simulink model "Current_Macchina3DOF"  (R2023a)
settings: Solver=VariableStepAuto  StartTime=0.0  StopTime=100  RelTol=1e-3
model workspace (MAT data in the model file):
  EngPwr = 352122.842504
  EngWc = 4.047
  Tdiff = 849
  Tlim = 1000
  VEH.Mass = 1181
  VEH.StaticNormalFrontLoad.FR = 264.666666667
  VEH.StaticNormalFrontLoad.FL = 264.666666667
  VEH.StaticNormalRearLoad.RR = 322
  VEH.StaticNormalRearLoad.RL = 322
  VEH.WheelBase = 3.075
  VEH.FrontAxlePositionfromCG = 1.515
  VEH.RearAxlePositionfromCG = 1.504
  VEH.HeightCG = 0.134
  VEH.FrontalArea = 2.11
  VEH.DragCoefficient = 0.33
  VEH.NumberOfWheelsPerAxle = 2
  VEH.Thread.FR = 1.705
  VEH.Thread.RR = 1.705
  VEH.PitchMomentInertia = 1922.66666667
  VEH.RollMomentInertia = 432.333333333
  VEH.YawMomentInertia = 2066
  VEH.SteeringRatio = 18
  VEH.TrackWidth = 1.922
  VEH.SprungMass = 1096.72266667
  VEH.InitialLongPosition = 0
  VEH.InitialLatPosition = 3.125
  VEH.InitialVertPosition = 0.0111
  VEH.InitialRollAngle = 0
  VEH.InitialPitchAngle = -0.000732
  VEH.InitialYawAngle = 0
  VEH.InitialLongVel = 0
  VEH.InitialLatVel = 0
  VEH.InitialVertVel = 0
  VEH.InitialRollRate = 0
  VEH.InitialPitchRate = 0
  VEH.InitialYawRate = 0
libraries: vehdynlibtirecommon x4, sim3dphyssensorlib x4, autolibutils x3, visionsinks x3, sim3dcameralib x2, sharedtransform x2, vehdynlibsteering x2, vehdynlibtire x1, sim3dlib x1, vdynlib x1, autolibshared x1
settings Model: Creator=gabri  LastModifiedBy=Luzi

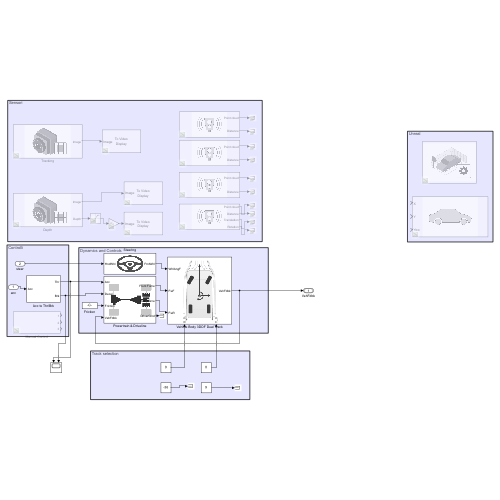
[thumbnail: Simulink's stored preview of the top-level diagram]
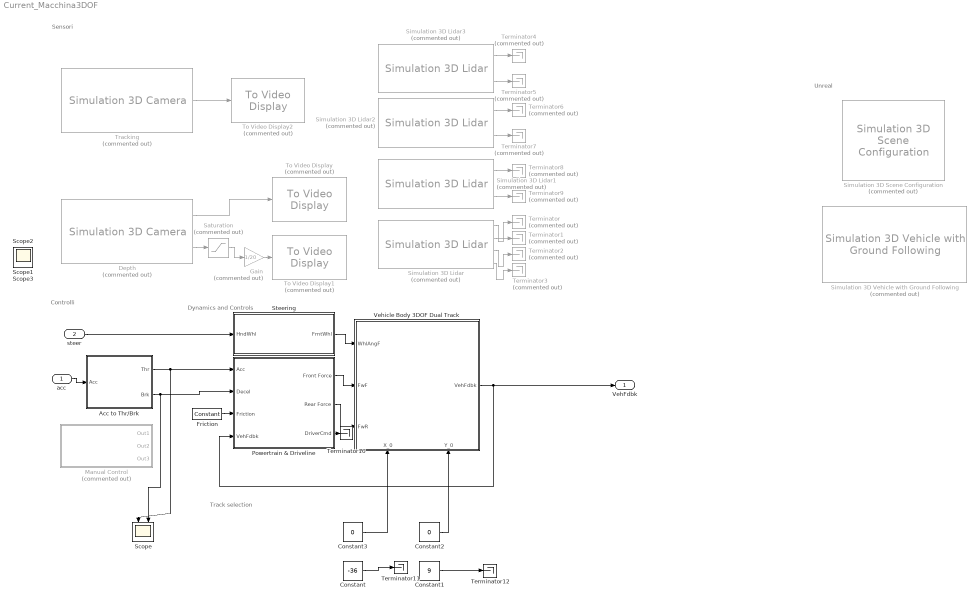
== system Current_Macchina3DOF ==
  note: Track selection
  note: Controlli
  note: Sensori
  note: Unreal
  note: Dynamics and Controls
  acc : Inport  LockScale=on
  steer : Inport  Port=2
  Acc to Thr/Brk : Subsystem
  Constant : Constant  Value=-36
  Constant1 : Constant  Value=9
  Constant2 : Constant  Value=0
  Constant3 : Constant  Value=0
  Depth : sim3dcameralib/Simulation 3D Camera  Priority=1  Commented=on  sensorTag=Sim3dSensor1  sensorId=1  sensorName=Sim3dSensor1  vehTagList={'Scene Origin';'SimulinkVehicle1'}  vehTag=SimulinkVehicle1  mountLoc=Origin  offsetFlag=on  tmountOffset=[-0.236, -0.01, 1.265]  extTmount=off  rmountOffset=[0, 0, 0]  extRmount=off  FocalLength=[643, 643]  OpticalCenter=[640, 360]  ImageSize=[720, 1280]  RadialDistortion=[0, 0]  TangentialDistortion=[0, 0]  SensorSkew=0  DepthOutportEnabled=on  SemanticOutportEnabled=off  TransformOutportEnabled=off  SampleTime=-1  mountPoint=[-0.236 0.01 1.265]  mountOrientation=[0 0 0]  aMode=3  ID=1
      settings: LibrarySourceBlock=drivingsim3d/Simulation 3D Camera
  Friction : vehdynlibtirecommon/Constant  const=0.8  numWheels=4
  Gain : Gain  Commented=on  Gain=1/20
  Manual Control : Subsystem  Commented=on
  Powertrain & Driveline : Subsystem
      mask Display: image('vdbslibpt.png');
  Saturation : Saturate  Commented=on  UpperLimit=20  LowerLimit=0
  Scope : Scope  NumInputPorts=2
  Simulation 3D Lidar : sim3dphyssensorlib/Simulation 3D Lidar  Priority=1  Commented=on  sensorTag=Sim3dSensor3  sensorId=3  sensorName=Sim3dSensor3  vehTagList={'Scene Origin';'SimulinkVehicle1'}  vehTag=SimulinkVehicle1  mountLoc=Origin  offsetFlag=on  tmountOffset=[1.52, -0.348, 0.12]  rmountOffset=[0, 0, 0]  DetectionRange=12  RangeResolution=0.01  VerticalFOV=2  VerticalResolution=2  HorizontalFOV=2  HorizontalResolution=0.54  DistanceOutportEnabled=on  ReflectivityOutportEnabled=off  SemanticOutportEnabled=off  TransformOutportEnabled=on  SampleTime=-1  mountPoint=[1.52 0.348 0.12]  mountOrientation=[0 0 0]  aMode=3  ID=3
      settings: LibrarySourceBlock=drivingsim3d/Simulation 3D Lidar
  Simulation 3D Lidar1 : sim3dphyssensorlib/Simulation 3D Lidar  Priority=1  Commented=on  sensorTag=Sim3dSensor4  sensorId=4  sensorName=Sim3dSensor4  vehTagList={'Scene Origin';'SimulinkVehicle1'}  vehTag=SimulinkVehicle1  mountLoc=Origin  offsetFlag=on  tmountOffset=[1.515, -0.393, 0.12]  rmountOffset=[0, 0, -22]  DetectionRange=12  RangeResolution=0.01  VerticalFOV=2  VerticalResolution=2  HorizontalFOV=2  HorizontalResolution=0.54  DistanceOutportEnabled=on  ReflectivityOutportEnabled=off  SemanticOutportEnabled=off  TransformOutportEnabled=off  SampleTime=-1  mountPoint=[1.515 0.393 0.12]  mountOrientation=[0 0 22]  aMode=3  ID=4
      settings: LibrarySourceBlock=drivingsim3d/Simulation 3D Lidar
  Simulation 3D Lidar2 : sim3dphyssensorlib/Simulation 3D Lidar  Priority=1  Commented=on  sensorTag=Sim3dSensor5  sensorId=5  sensorName=Sim3dSensor5  vehTagList={'Scene Origin';'SimulinkVehicle1'}  vehTag=SimulinkVehicle1  mountLoc=Origin  offsetFlag=on  tmountOffset=[1.52, 0.348, 0.12]  rmountOffset=[0, 0, 0]  DetectionRange=12  RangeResolution=0.01  VerticalFOV=2  VerticalResolution=2  HorizontalFOV=2  HorizontalResolution=0.54  DistanceOutportEnabled=on  ReflectivityOutportEnabled=off  SemanticOutportEnabled=off  TransformOutportEnabled=off  SampleTime=-1  mountPoint=[1.52 -0.348 0.12]  mountOrientation=[0 0 0]  aMode=3  ID=5
      settings: LibrarySourceBlock=drivingsim3d/Simulation 3D Lidar
  Simulation 3D Lidar3 : sim3dphyssensorlib/Simulation 3D Lidar  Priority=1  Commented=on  sensorTag=Sim3dSensor6  sensorId=6  sensorName=Sim3dSensor6  vehTagList={'Scene Origin';'SimulinkVehicle1'}  vehTag=SimulinkVehicle1  mountLoc=Origin  offsetFlag=on  tmountOffset=[1.515, 0.393, 0.12]  rmountOffset=[0, 0, 22]  DetectionRange=12  RangeResolution=0.01  VerticalFOV=2  VerticalResolution=2  HorizontalFOV=2  HorizontalResolution=0.54  DistanceOutportEnabled=on  ReflectivityOutportEnabled=off  SemanticOutportEnabled=off  TransformOutportEnabled=off  SampleTime=-1  mountPoint=[1.515 -0.393 0.12]  mountOrientation=[0 0 -22]  aMode=3  ID=6
      settings: LibrarySourceBlock=drivingsim3d/Simulation 3D Lidar
  Simulation 3D Scene Configuration : sim3dlib/Simulation 3D Scene Configuration  Priority=0  Commented=on  ProjectFormat=Unreal Editor  SceneDesc=Straight road  ProjectName=D:\MATLAB\toolbox\shared\sim3d_projects\automotive_project\UE4\WindowsNoEditor\VehicleSimulation.exe  ScenePath=/Game/Maps/HwStrght  UEProjPath=C:\Users\gabriele\Documents\Unreal Projects\4_27\FSAE\RT3D\RT3D.uproject  EnableOpenDRIVE=off  vehTagList={'Scene Origin';'SimulinkVehicle1'}  vehTag=SimulinkVehicle1  OpVisEn=off  Ts=.01  EnableWindow=on  EnableRemoteAccess=off  EnableWeather=off  SunAltitude=40.0  SunAzimuth=90  clouds=10  wind=1  fog=0  rain=0  EnableGeospatial=off  OriginHeight=200  OriginLatitude=40.744652  OriginLongitude=-73.988864  MapStyle=Aerial  AdditionalAssetIDs=[]  UseAdvancedSunSky=off  SolarTime=11  TimeZone=-5  Day=21  Month=9  Year=2022  UseDaylightSavingTime=on  DSTStartDay=10  DSTStartMonth=3  DSTEndDay=3  DSTEndMonth=11  DSTSwitchHour=2  sensorTag=MainCamera1  sensorId=1  sensorName=MainCamera1  mountLoc=Origin  offsetFlag=off  tmountOffset=[0, 0, 0]  rmountOffset=[0, 0, 0]  HorizontalResolution=1280  VerticalResolution=720  HorizontalFOV=60  mountPoint=[0 0 0]  mountOrientation=[0 0 0]  aMode=2  ID=1  GeoTrigger=Inactive
      settings: LibrarySourceBlock=vdynlib/Vehicle Scenarios/Sim3D/Sim3D Core/Simulation 3D Scene Configuration
  Simulation 3D Vehicle with Ground Following : vdynlib/Vehicle Scenarios/Sim3D/Sim3D Vehicle/Components/Simulation 3D Vehicle with Ground Following  Priority=-1  Commented=on  PassVehMesh=Custom  MeshPath=/Game/Car1/FC_Model.FC_Model  TrackWidth=1.4  WheelBase=3  WheelRadius=0.35  VehColor=Red  InitialPos=[0, 0, 0]  InitialRot=[0, 0, 0]  ActorName=SimulinkVehicle1  VehLightsControl=off  HeadlightColor=[ 1, 1, 1 ]  HighBeamIntensity=100000  LowBeamIntensity=60000  HighBeamConeAngle=1.22  LowBeamConeAngle=1.22  LeftHeadlightOrientation=[ 0, 0 ]  RightHeadlightOrientation=[ 0, 0 ]  BrakelightIntensity=200  ReverselightIntensity=500  SignallightIntensity=500  SignallightPeriod=1  SignalPulseWidth=50  SampleTime=-1  ActorType=SimulinkVehicle  ID=1  aMode=2  ActorTag=SimulinkVehicle1  CoordinateScheme=SAE
  Steering : Subsystem
      mask Display: image('vdbslibsteer.png');
  Terminator{,1..9} (10 alike) : Terminator  Commented=on
  Terminator10 : Terminator
  Terminator11 : Terminator
  Terminator12 : Terminator
  To Video Display : visionsinks/To Video Display  Commented=on  windowSizeMode=Normal  openAtMdlStart=on  fullScreen=off  videoWindowX=536805376  videoWindowY=536805376  saveWindowSize=off  videoWindowWidth=2147483647  videoWindowHeight=2147483647  inputColorFormat=RGB  inputType=Obsolete  imagePorts=One multidimensional signal  OutputDevice=On-screen video monitor  dataOrg=Column-major  isWindowOpen=off
  To Video Display1 : visionsinks/To Video Display  Commented=on  windowSizeMode=Normal  openAtMdlStart=on  fullScreen=off  videoWindowX=536805376  videoWindowY=536805376  saveWindowSize=off  videoWindowWidth=2147483647  videoWindowHeight=2147483647  inputColorFormat=RGB  inputType=Obsolete  imagePorts=One multidimensional signal  OutputDevice=On-screen video monitor  dataOrg=Column-major  isWindowOpen=off
  To Video Display2 : visionsinks/To Video Display  Commented=on  windowSizeMode=Normal  openAtMdlStart=on  fullScreen=off  videoWindowX=536805376  videoWindowY=536805376  saveWindowSize=off  videoWindowWidth=2147483647  videoWindowHeight=2147483647  inputColorFormat=RGB  inputType=Obsolete  imagePorts=One multidimensional signal  OutputDevice=On-screen video monitor  dataOrg=Column-major  isWindowOpen=off
  Tracking : sim3dcameralib/Simulation 3D Camera  Priority=1  Commented=on  sensorTag=Sim3dSensor2  sensorId=2  sensorName=Sim3dSensor2  vehTagList={'Scene Origin';'SimulinkVehicle1'}  vehTag=SimulinkVehicle1  mountLoc=Origin  offsetFlag=on  tmountOffset=[0.855, 0, 0.655]  extTmount=off  rmountOffset=[0, 0, 0]  extRmount=off  FocalLength=[643, 643]  OpticalCenter=[640, 360]  ImageSize=[720, 1280]  RadialDistortion=[0, 0]  TangentialDistortion=[0, 0]  SensorSkew=0  DepthOutportEnabled=off  SemanticOutportEnabled=off  TransformOutportEnabled=off  SampleTime=-1  mountPoint=[0.855 0 0.655]  mountOrientation=[0 0 0]  aMode=3  ID=2
      settings: LibrarySourceBlock=drivingsim3d/Simulation 3D Camera
  Vehicle Body 3DOF Dual Track : Subsystem
      settings: PortSchema="{\"entries\":[{\"content\":{\"sides\":[{\"content\":{\"connectorIds\":[\"In1\",\"In2\",\"In3\"]},\"type\":\"ConnectorPlacement.EquallySpacedRectSide\",\"uuid\":\"4036215f-6a7b-43f4-bf3a-9e74b907d558\"},{\"content\":{\"connectorIds\":[\"Out1\"],\"side\":\"RIGHT\"},\"type\":\"ConnectorPlacement.EquallySpacedRectSide\",\"uuid\":\"eff6a8c4-1212-4912-9320-06419e317e63\"},{\"content\":{\"side\":\"TOP\"},\"type\":\"ConnectorPlacement.EquallySpacedRectSide\",\"uuid\":\"7c86d461-eb08-4ad0-9f05-3e331398aa8b\"},{\"content\":{\"connectorIds\":[\"In4\",\"In5\"],\"side\":\"BOTTOM\"},\"type\":\"ConnectorPlacement.EquallySpacedRectSide\",\"uuid\":\"b22d0b58-a589-4aa7-a626-c5ccf618b747\"}]},\"type\":\"ConnectorPlacement.EquallySpacedConnector\",\"uuid\":\"19937682-2ace-470e-aa72-0faa8a79652b\"}],\"packageUris\":[\"http://schema.mathworks.com/mf0/Connector/R2020b\"],\"version\":\"1.0\"}"
      mask Display: image('3dofdtrack.png');
  VehFdbk : Outport  OutDataTypeStr=Bus: VehFdbk
  Scope1 : Scope
  Scope2 : Scope
  Scope3 : Scope
  wires:
  Powertrain & Driveline/2(Rear Force) -> Vehicle Body 3DOF Dual Track/3(FwR)
  Steering/1(FrntWhl) -> Vehicle Body 3DOF Dual Track/1(WhlAngF)
  Powertrain & Driveline/1(Front Force) -> Vehicle Body 3DOF Dual Track/2(FwF)
  Friction/1 -> Powertrain & Driveline/3(Friction)
  Depth/2 -> Saturation/1
  Depth/1 -> To Video Display/1
  Saturation/1 -> Gain/1
  Gain/1 -> To Video Display1/1
  Simulation 3D Lidar/1 -> Terminator/1
  Simulation 3D Lidar/2 -> Terminator1/1
  Constant/1 -> Terminator11/1
  Constant1/1 -> Terminator12/1
  Simulation 3D Lidar/3 -> Terminator2/1
  Simulation 3D Lidar/4 -> Terminator3/1
  Constant2/1 -> Vehicle Body 3DOF Dual Track/5(Y_0)
  Tracking/1 -> To Video Display2/1
  Simulation 3D Lidar3/1 -> Terminator4/1
  Simulation 3D Lidar3/2 -> Terminator5/1
  Simulation 3D Lidar2/1 -> Terminator6/1
  Simulation 3D Lidar2/2 -> Terminator7/1
  Simulation 3D Lidar1/1 -> Terminator8/1
  Simulation 3D Lidar1/2 -> Terminator9/1
  Constant3/1 -> Vehicle Body 3DOF Dual Track/4(X_0)
  Vehicle Body 3DOF Dual Track/1(VehFdbk) -> Powertrain & Driveline/4(VehFdbk), VehFdbk/1
  Powertrain & Driveline/3(DriverCmd) -> Terminator10/1
  acc/1 -> Acc to Thr/Brk/1(Acc)
  Acc to Thr/Brk/1(Thr) -> Scope/1, Powertrain & Driveline/1(Acc)
  Acc to Thr/Brk/2(Brk) -> Powertrain & Driveline/2(Decel), Scope/2
  steer/1 -> Steering/1(HndWhl)

== system Current_Macchina3DOF/Acc to Thr//Brk ==
  Acc : Inport
  Switch1 : Switch  Criteria=u2 > Threshold  SaturateOnIntegerOverflow=off  InputSameDT=off
  Switch2 : Switch  Criteria=u2 > Threshold  SaturateOnIntegerOverflow=off  InputSameDT=off
  Unary Minus : UnaryMinus
  Zero : Constant  Value=0  OutDataTypeStr=Inherit: Inherit via back propagation
  Zero1 : Constant  Value=0  OutDataTypeStr=Inherit: Inherit via back propagation
  Thr : Outport
  Brk : Outport  Port=2
  wires:
  Acc/1 -> Switch1/1, Switch1/2, Unary Minus/1, Switch2/2
  Zero1/1 -> Switch1/3
  Switch1/1 -> Thr/1
  Zero/1 -> Switch2/1
  Unary Minus/1 -> Switch2/3
  Switch2/1 -> Brk/1

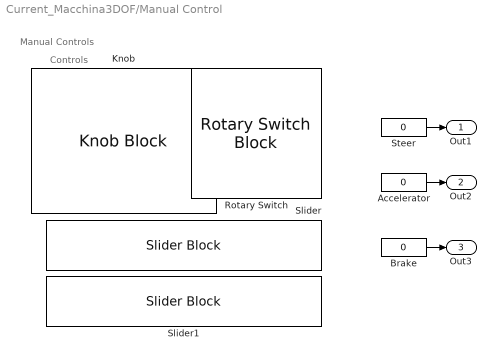
== system Current_Macchina3DOF/Manual Control ==
  note: Manual Controls
  note: Controls
  Accelerator : Constant  Value=0  SampleTime=-1
  Brake : Constant  Value=0  SampleTime=-1
  Knob : KnobBlock  LabelPosition=Bottom  ScaleMin=-90  ScaleMax=90  TickInterval=30
  Rotary Switch : RotarySwitchBlock  LabelPosition=Bottom
      settings: Values={{'R', 'N', 'D'}, [-1 0 1]}
  Slider : SliderBlock  LabelPosition=Bottom  ScaleMax=1  TickInterval=.2
  Slider1 : SliderBlock  LabelPosition=Bottom  ScaleMax=1  TickInterval=.2
  Steer : Constant  Value=0  SampleTime=-1
  Out1 : Outport
  Out2 : Outport  Port=2
  Out3 : Outport  Port=3
  wires:
  Steer/1 -> Out1/1
  Brake/1 -> Out3/1
  Accelerator/1 -> Out2/1

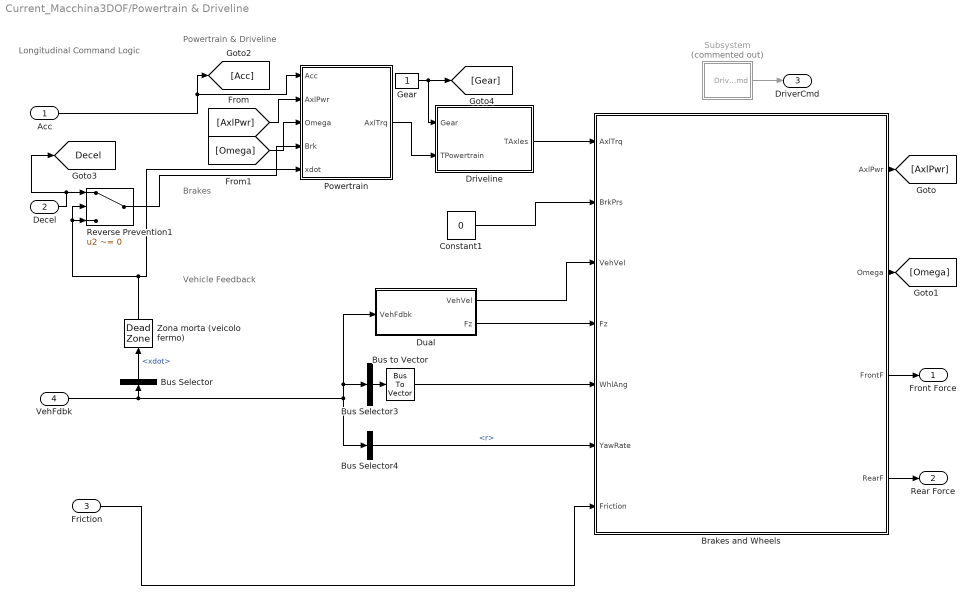
== system Current_Macchina3DOF/Powertrain & Driveline ==
  note: Longitudinal Command Logic
  note: Brakes
  note: Powertrain & Driveline
  note: Vehicle Feedback
  Acc : Inport
  Decel : Inport  Port=2
  Friction : Inport  Port=3
  VehFdbk : Inport  Port=4
  Brakes and Wheels : Subsystem  TreatAsAtomicUnit=on
      mask Display: image('vdbslibwhls.png');
  Bus Selector : BusSelector  OutputSignals=BdyFrm.Cg.Vel.xdot
  Bus Selector3 : BusSelector  OutputSignals=BdyFrm.FrntAxl.Steer.WhlAngFL,BdyFrm.FrntAxl.Steer.WhlAngFR,BdyFrm.RearAxl.Steer.WhlAngRL,BdyFrm.RearAxl.Steer.WhlAngRR  OutputAsBus=on
  Bus Selector4 : BusSelector  OutputSignals=BdyFrm.Cg.AngVel.r
  Bus to Vector : BusToVector
  Constant1 : Constant  Value=0
  Driveline : Subsystem  Variant=on  VariantControlMode=label  VariantControl=Variant1  LabelModeActiveChoice=0
  Dual : Subsystem  VariantControl=1
  Gear : Constant
  Powertrain : Subsystem
  Reverse Prevention1 : Switch  Criteria=u2 ~= 0  SaturateOnIntegerOverflow=off  InputSameDT=off
  Subsystem : Subsystem  Commented=on
  Zona morta (veicolo fermo) : DeadZone  LowerValue=-0.3  UpperValue=0.0002
  Front Force : Outport  VectorParamsAs1DForOutWhenUnconnected=off
  Rear Force : Outport  Port=2  VectorParamsAs1DForOutWhenUnconnected=off
  DriverCmd : Outport  Port=3  VectorParamsAs1DForOutWhenUnconnected=off
  tag scope: Decel=global
  wires:
  Bus Selector3/1 -> Bus to Vector/1
  Acc/1 -> [Acc], Powertrain/1(Acc)
  Powertrain/1(AxlTrq) -> Driveline/2(TPowertrain)
  [AxlPwr] -> Powertrain/2(AxlPwr)
  [Omega] -> Powertrain/3(Omega)
  Gear/1 -> Driveline/1(Gear), [Gear]
  Friction/1 -> Brakes and Wheels/7(Friction)
  Brakes and Wheels/2(Omega) -> [Omega]
  Brakes and Wheels/3(FrontF) -> Front Force/1
  Brakes and Wheels/4(RearF) -> Rear Force/1
  Brakes and Wheels/1(AxlPwr) -> [AxlPwr]
  Bus to Vector/1 -> Brakes and Wheels/5(WhlAng)
  Dual/2(Fz) -> Brakes and Wheels/4(Fz)
  Bus Selector4/1 -> Brakes and Wheels/6(YawRate)  "<r>"
  Constant1/1 -> Brakes and Wheels/2(BrkPrs)
  Driveline/1(TAxles) -> Brakes and Wheels/1(AxlTrq)
  Dual/1(VehVel) -> Brakes and Wheels/3(VehVel)
  Subsystem/1(DriverCmd) -> DriverCmd/1
  VehFdbk/1 -> Bus Selector/1, Dual/1(VehFdbk), Bus Selector3/1, Bus Selector4/1
  Decel/1 -> Reverse Prevention1/1, [Decel]
  Bus Selector/1 -> Zona morta (veicolo fermo)/1  "<xdot>"
  Zona morta (veicolo fermo)/1 -> Reverse Prevention1/3, Reverse Prevention1/2, Powertrain/5(xdot)
  Reverse Prevention1/1 -> Powertrain/4(Brk)

== system Current_Macchina3DOF/Steering ==
  HndWhl : Inport
  Kinematic Steering : vehdynlibsteering/Kinematic Steering  Commented=on  StrgType=Rack and pinion  StrgRatioType=Constant  Loc=Front  NrmlFctr=0.01  TrckWdth=1.10  WhlBase=1.524  Db=0  StrgRng=5/6*pi  StrgAngBpts="[-6.2832   -5.0265   -3.7699   -2.5133   -1.2566         0    1.2566    2.5133    3.7699    5.0265    6.2832]"  StrgRatioTbl=|  StrgRatio=100  PctAckIn=off  PctAck=100  PctAckTbl=ones(1,11)*100  StrgArmLngth=0.313  RckCsLngth=0.517  TieRodLngth=0.00001  D=0.1024  PnnRadius=0.07  PnnRadiusTbl="[0.0055    0.0055    0.0056    0.0057    0.0058    0.0057    0.0057    0.0057    0.0056    0.0055    0.0055]"  RodLngth=0.1  ParaArmLngth=0.9  aMode=2
      | [13.5000   13.3750   13.2500   13.1250   13.0000   13.0000   13.0000   13.1250   13.2500   13.3750   13.5000
      | ]
  Kinematic Steering1 : vehdynlibsteering/Kinematic Steering  StrgType=Parallel  StrgRatioType=Constant  Loc=Front  NrmlFctr=0.01  TrckWdth=1.10  WhlBase=1.524  Db=0  StrgRng=5/6*pi  StrgAngBpts="[-6.2832   -5.0265   -3.7699   -2.5133   -1.2566         0    1.2566    2.5133    3.7699    5.0265    6.2832]"  StrgRatioTbl=|  StrgRatio=5  PctAckIn=off  PctAck=100  PctAckTbl=ones(1,11)*100  StrgArmLngth=0.313  RckCsLngth=0.517  TieRodLngth=0.00001  D=0.1024  PnnRadius=0.07  PnnRadiusTbl="[0.0055    0.0055    0.0056    0.0057    0.0058    0.0057    0.0057    0.0057    0.0056    0.0055    0.0055]"  RodLngth=0.1  ParaArmLngth=0.9  aMode=2
      | [13.5000   13.3750   13.2500   13.1250   13.0000   13.0000   13.0000   13.1250   13.2500   13.3750   13.5000
      | ]
  Mux : Mux  Inputs=2
  Signal Specification : SignalSpecification  Unit=deg
  Terminator : Terminator
  Terminator6 : Terminator
  Unit Conversion : UnitConversion
  FrntWhl : Outport  VectorParamsAs1DForOutWhenUnconnected=off
  wires:
  Signal Specification/1 -> Unit Conversion/1
  Kinematic Steering/1 -> Terminator6/1
  HndWhl/1 -> Signal Specification/1
  Unit Conversion/1 -> Kinematic Steering1/1
  Mux/1 -> FrntWhl/1
  Kinematic Steering1/3 -> Mux/2
  Kinematic Steering1/2 -> Mux/1
  Kinematic Steering1/1 -> Terminator/1

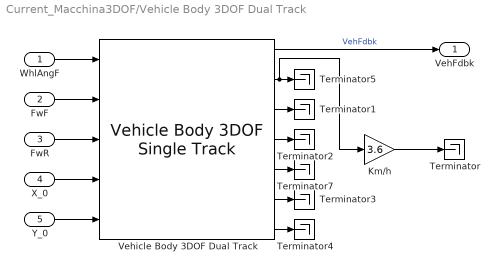
== system Current_Macchina3DOF/Vehicle Body 3DOF Dual Track ==
  WhlAngF : Inport
  FwF : Inport  Port=2
  FwR : Inport  Port=3
  X_0 : Inport  Port=4
  Y_0 : Inport  Port=5
  Km/h : Gain  Gain=3.6
  Terminator{,1..5,7} (7 alike) : Terminator
  Vehicle Body 3DOF Dual Track : autolibshared/Vehicle Body 3DOF Single Track  trackMode=Dual  inputMode=External forces  frontSteerMode=on  rearSteerMode=off  windMode=off  muMode=off  extFMode=off  extMMode=off  htchFMode=off  htchMMode=off  extXo=on  extpsio=off  extxdoto=off  extro=off  extYo=on  extTamb=off  extydoto=off  aMode=2  NF=2  NR=2  m=256+60  a=1  b=0.6  h=0.35  dh=1  hh=0.2  X_o=-36  xdot_o=0  CalphaMode=off  sigmaMode=on  d=0  hl=0  w=[1.4,1.4]  Cy_f=12e3  Cy_r=11e3  sigma_f=.1  sigma_r=.1  alpha_f_brk=[-.1 .1]  Cy_f_data=[-9e3 9e3]  alpha_r_brk=[-.1 .1]  Cy_r_data=[-9e3 9e3]  Y_o=9  ydot_o=0  Izz=250  psi_o=0  r_o=0  Af=1.194  Cd=1.124  Cl=1.531  Cpm=.1  beta_w=[0:0.02:0.3]  Cs=[0:0.06:0.9]  Cym=[0:0.02:0.3]  Pabs=101325  Tair=273  g=9.81  mu=1  xdot_tol=.1  Fznom=5000  Fxtire_sat=7e4  Fytire_sat=7e4  longOff=0  latOff=0  vertOff=0  wrapAng=on
  VehFdbk : Outport
  wires:
  Vehicle Body 3DOF Dual Track/6 -> Terminator3/1
  Vehicle Body 3DOF Dual Track/2 -> Km/h/1, Terminator5/1
  Vehicle Body 3DOF Dual Track/3 -> Terminator1/1
  Vehicle Body 3DOF Dual Track/4 -> Terminator2/1
  Vehicle Body 3DOF Dual Track/7 -> Terminator4/1
  Vehicle Body 3DOF Dual Track/1 -> VehFdbk/1  "VehFdbk"
  Vehicle Body 3DOF Dual Track/5 -> Terminator7/1
  FwF/1 -> Vehicle Body 3DOF Dual Track/2
  WhlAngF/1 -> Vehicle Body 3DOF Dual Track/1
  FwR/1 -> Vehicle Body 3DOF Dual Track/3
  X_0/1 -> Vehicle Body 3DOF Dual Track/4
  Y_0/1 -> Vehicle Body 3DOF Dual Track/5
  Km/h/1 -> Terminator/1

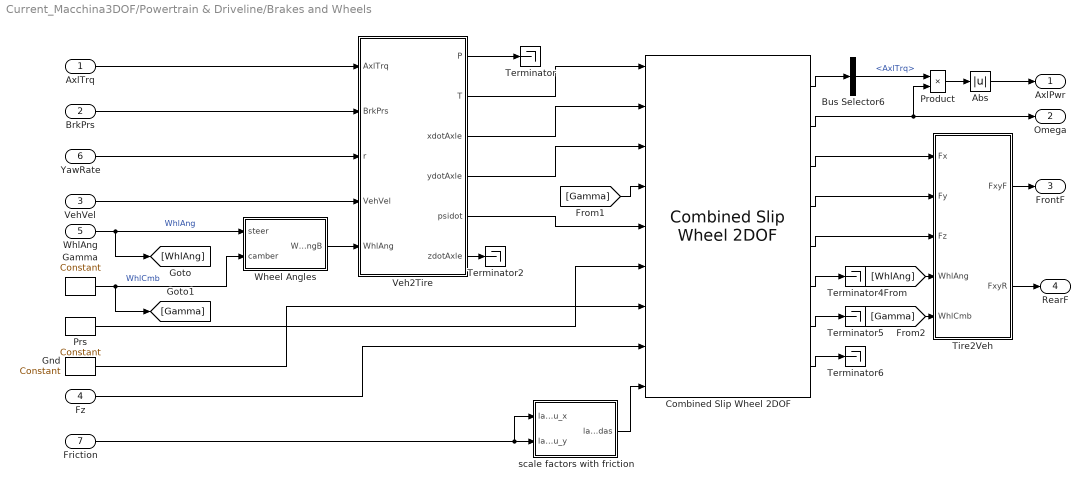
== system Current_Macchina3DOF/Powertrain & Driveline/Brakes and Wheels ==
  AxlTrq : Inport
  BrkPrs : Inport  Port=2
  VehVel : Inport  Port=3
  Fz : Inport  Port=4  PortDimensions=4
  WhlAng : Inport  Port=5
  YawRate : Inport  Port=6
  Friction : Inport  Port=7
  Abs : Abs  SaturateOnIntegerOverflow=off
  Bus Selector6 : BusSelector  OutputSignals=AxlTrq
  Combined Slip Wheel 2DOF : vehdynlibtire/Combined Slip Wheel 2DOF  tireType=External file  BrakeType=None  vertType=None  plySteer=off  turnslip=off  mu_static=.3  mu_kinetic=.2  disk_abore=.05  Rm=.177  num_pads=2  drum_abore=0.0508  drum_a=0.123  drum_c=0.212  drum_r=0.15  drum_theta1=0  drum_theta2=126  brake_p_bpt=[1 11.4736842105263 21.9473684210526 32.4210526315789 42.8947368421053 53.3684210526316 63.8421052631579 74.3157894736842 84.7894736842105 95.2631578947368 105.736842105263 116.210526315789 126.684210526316 137.157894736842 147.631578947368 158.105263157895 168.578947368421 179.052631578947 189.526315789474 200]  brake_n_bpt=[0 52.6315789473684 105.263157894737 157.894736842105 210.526315789474 263.157894736842 315.789473684211 368.421052631579 421.052631578947 473.684210526316 526.315789473684 578.947368421053 631.578947368421 684.210526315789 736.842105263158 789.473684210526 842.105263157895 894.736842105263 947.368421052632 1000]  f_brake_t=[43.4900602404453 42.5056030554862 41.5350898940194 40.5780454442085 39.6340111501808 38.7025443887544 37.7832176914519 36.8756180088306 35.9793460143796 35.0940154454303 34.2192524787115 33.3546951383474 32.4999927342521 31.6548053290159 30.8188032315107 29.991666515561 29.1730845621415 28.362755623661 27.5603864089927 26.765691687993;498.991217495636 487.695866636631 476.560505099801 465.579679307235 454.748127933653 444.060772460445 433.51270824929 423.099196101319 412.81565427025 402.657650900201 392.620896861006 382.701238955775 372.894653477208 363.197240090814 353.605216024701 344.114910546964 334.722759712992 325.425301366216 316.219170376863 307.10109410434;954.492374750826 932.886130217776 911.585920305583 890.581313170261 869.862244717126 849.419000532136 829.242198807128 809.322774193808 789.651962526121 770.221286354971 751.0225412433 732.047782773203 713.289314220164 694.739674852612 676.391628817892 658.238154578366 640.272434863842 622.48784710877 604.877954344734 587.436496520688;1409.99353200602 1378.07639379892 1346.61133551136 1315.58294703329 1284.9763615006 1254.77722860383 1224.97168936497 1195.5463522863 1166.48827078199 1137.78492180974 1109.42418562559 1081.39432659063 1053.68397496312 1026.28210961441 999.178041611083 972.361398609768 945.822110014692 919.550392851325 893.536738312604 867.771898937035;1865.49468926121 1823.26665738007 1781.63675071715 1740.58458089631 1700.09047828407 1660.13545667552 1620.7011799228 1581.76993037878 1543.32457903786 1505.34855726451 1467.82583000789 1430.74087040806 1394.07863570608 1357.82454437621 1321.96445440427 1286.48464264117 1251.37178516554 1216.61293859388 1182.19552228048 1148.10730135338;2320.9958465164 2268.45692096121 2216.66216592293 2165.58621475934 2115.20459506754 2065.49368474721 2016.43067048064 1967.99350847127 1920.16088729373 1872.91219271928 1826.22747439018 1780.08741422549 1734.47329644903 1689.36697913801 1644.75086719747 1600.60788667257 1556.92146031639 1513.67548433643 1470.85430624835 1428.44270376973;2776.49700377159 2713.64718454235 2651.68758112871 2590.58784862237 2530.31871185102 2470.8519128189 2412.16016103848 2354.21708656376 2296.9971955496 2240.47582817405 2184.62911877248 2129.43395804292 2074.86795719199 2020.9094138998 1967.53727999066 1914.73113070398 1862.47113546724 1810.73803007899 1759.51309021622 1708.77810618608;3231.99816102678 3158.8374481235 3086.71299633449 3015.58948248539 2945.43282863449 2876.21014089059 2807.88965159632 2740.44066465625 2673.83350380547 2608.03946362882 2543.03076315477 2478.78050186034 2415.26261793494 2352.4518486616 2290.32369278385 2228.85437473538 2168.02081061809 2107.80057582154 2048.17187418409 1989.11350860242;3687.49931828197 3604.02771170464 3521.73841154027 3440.59111634842 3360.54694541796 3281.56836896228 3203.61914215416 3126.66424274874 3050.66981206134 2975.60309908359 2901.43240753707 2828.12704567777 2755.6572786779 2683.9942834234 2613.11010557704 2542.97761876678 2473.57048576894 2404.8631215641 2336.83065815196 2269.44891101877;4143.00047553716 4049.21797528579 3956.76382674606 3865.59275021144 3775.66106220143 3686.92659703397 3599.34863271199 3512.88782084123 3427.50612031721 3343.16673453836 3259.83405191936 3177.4735894952 3096.05193942085 3015.5367181852 2935.89651837023 2857.10086279818 2779.12016091979 2701.92566730665 2625.48944211983 2549.78431343512;4598.50163279235 4494.40823886693 4391.78924195184 4290.59438407447 4190.77517898491 4092.28482510566 3995.07812326983 3899.11139893372 3804.34242857308 3710.73036999313 3618.23569630166 3526.82013331263 3436.44660016381 3347.079152947 3258.68293116342 3171.22410682959 3084.66983607064 2998.98821304921 2914.1482260877 2830.11971585147;5054.00279004754 4939.59850244808 4826.81465715762 4715.59601793749 4605.88929576838 4497.64305317735 4390.80761382767 4285.3349770262 4181.17873682896 4078.2940054479 3976.63734068395 3876.16667713006 3776.84126090677 3678.62158770879 3581.46934395661 3485.34735086099 ...(+2764 chars)]  tireParamSet=C:\Users\gabri\Documents\MATLAB\Macchina 3DOF\File Tir\Round_6_Hoosier_R25B_20p5x7_13_on_7in\Prova_tagli.tir  PRESMAX=1000000  PRESMIN=10000  FZMAX=1500  FZMIN=100  VXLOW=1  KPUMAX=0.25  KPUMIN=-0.25  ALPMAX=0.26  ALPMIN=-0.26  CAMMAX=0.17453  CAMMIN=-0.17453  LONGVL=11.1976  FxRelFreqLwrLim=200*pi  FyRelFreqLwrLim=200*pi  MyRelFreqLwrLim=100*pi  omegao=0  br=1e-3  UNLOADED_RADIUS=0.2603  NOMPRES=56000  FNOMIN=1112  WIDTH=0.1778  RIM_RADIUS=0.1651  MASS=11.2  IYY=1.084  GRAVITY=-9.81  zo=0  zdoto=0  BREFF=0  DREFF=0  FREFF=0  Q_RE0=1.003  Q_V1=0.000864  Q_V2=0.025807  Q_FZ1=0  Q_FZ2=51.51  Q_FZ3=0  Q_FCX=0  Q_FCY=0  Q_FCY2=0  PFZ1=1  VERTICAL_STIFFNESS=93518  VERTICAL_DAMPING=189.709  BOTTOM_OFFST=0.01  BOTTOM_STIFF=2000000  LONGITUDINAL_STIFFNESS=505632.6  LATERAL_STIFFNESS=219162.7  PCFX1=-0.12193  PCFX2=0  PCFX3=0  PCFY1=-0.17034  PCFY2=0  PCFY3=0  Q_RA1=0.602  Q_RA2=1.024  Q_RB1=1.1137  Q_RB2=-0.09748  PCX1=1.29281  PDX1=2.85291  PDX2=-0.194993  PDX3=12.3297  PEX1=-0.462105  PEX2=0  PEX3=0.243755  PEX4=0.949647  PKX1=59.3779  PKX2=31.7365  PKX3=-0.978984  PHX1=0.00152312  PHX2=-0.00148338  PVX1=-0.125737  PVX2=-0.0612927  PPX1=0  PPX2=0  PPX3=0  PPX4=0  RBX1=19.0357  RBX2=10.4128  RBX3=0  RCX1=1.06651  REX1=0.333333  REX2=0.333333  RHX1=-0.0109476  QSX1=-0.00443732  QSX2=-1.6581  QSX3=0.0306188  QSX4=0.999998  QSX5=-0.999999  QSX6=0.633486  QSX7=-4.53259  QSX8=-3.99998  QSX9=-0.0141022  QSX10=1  QSX11=2.01193  QSX12=0  QSX13=0  QSX14=0  PPMX1=0  PCY1=1.47427  PDY1=-2.54738  PDY2=0.65  PDY3=2  PEY1=-0.145232  PEY2=-0.347662  PEY3=0.920215  PEY4=1  PEY5=0  PKY1=-42.4369  PKY2=1.11575  PKY3=1.3203  PKY4=1.8092  PKY5=0  PKY6=-1.1028  PKY7=-0.4695  PHY1=-0.000901398  PHY2=-0.000665924  PVY1=0.0150137  PVY2=0.0323928  PVY3=2.1464  PVY4=-3.18483  PPY1=0  PPY2=0  PPY3=0  PPY4=0  PPY5=0  RBY1=14.6663  RBY2=10.4  RBY3=-0.0198478  RBY4=0  RCY1=1.03616  REY1=-0.278673  REY2=-1.3708  RHY1=0.0150708  RHY2=0.0250437  RVY1=0.01  RVY2=-0.00871487  RVY3=0.0554968  RVY4=10.3162  RVY5=-1.39968  RVY6=22  QSY1=0  QSY2=0  QSY3=0  QSY4=0  QSY5=0  QSY6=0  QSY7=0  QSY8=0  QBZ1=9.19193  QBZ2=-6.4205  QBZ3=-12.3231  QBZ4=2.3916  QBZ5=-3.338  QBZ6=0  QBZ9=0  QBZ10=-0.3276  QCZ1=1.20276  QDZ1=0.177429  QDZ2=-0.0891027  QDZ3=1.1459  QDZ4=-22.3675  QDZ6=0.00624081  QDZ7=0.0183905  QDZ8=-0.856  QDZ9=-0.1181  QDZ10=0  QDZ11=0  QEZ1=-1.68588  QEZ2=0.317552  QEZ3=1.79338  QEZ4=0.190377  QEZ5=-10  QHZ1=-0.000110722  QHZ2=0.00242714  QHZ3=-0.05  QHZ4=-0.0696  PPZ1=0  PPZ2=0  SSZ1=-0.0628088  SSZ2=-0.0437683  SSZ3=0.980918  SSZ4=-0.615016  PDXP1=0.4  PDXP2=0  PDXP3=0  PKYP1=0.9786  PDYP1=0.4  PDYP2=0  PDYP3=0  PDYP4=0  PHYP1=1  PHYP2=0.15  PHYP3=0  PHYP4=-4  PECP1=0.49516  PECP2=2.5522e-06  QDTP1=10  QCRP1=0.12649  QCRP2=0.1  QBRP1=0.1  QDRP1=1  QDRP2=0  aMode=2
  Gamma : vehdynlibtirecommon/Constant  const=0  numWheels=4
  Gnd : vehdynlibtirecommon/Constant  const=0  numWheels=4
  Product : Product
  Prs : vehdynlibtirecommon/Constant  const=2.4e5  numWheels=4
  Terminator{,2,4..6} (5 alike) : Terminator
  Tire2Veh : Subsystem
  Veh2Tire : Subsystem
  Wheel Angles : Subsystem
  scale factors with friction : Subsystem  mask{numWheels=4}
      mask prompts: numWheels "Number of wheels"
  AxlPwr : Outport
  Omega : Outport  Port=2
  FrontF : Outport  Port=3
  RearF : Outport  Port=4
  wires:
  Gnd/1 -> Combined Slip Wheel 2DOF/7
  Combined Slip Wheel 2DOF/1 -> Bus Selector6/1
  Combined Slip Wheel 2DOF/2 -> Omega/1, Product/2
  Combined Slip Wheel 2DOF/7 -> Terminator5/1
  Combined Slip Wheel 2DOF/6 -> Terminator4/1
  Product/1 -> Abs/1
  Fz/1 -> Combined Slip Wheel 2DOF/8
  Veh2Tire/3(xdotAxle) -> Combined Slip Wheel 2DOF/2
  Combined Slip Wheel 2DOF/8 -> Terminator6/1
  Prs/1 -> Combined Slip Wheel 2DOF/6
  Friction/1 -> scale factors with friction/1(lamda_mu_x), scale factors with friction/2(lamda_mu_y)
  Abs/1 -> AxlPwr/1
  Bus Selector6/1 -> Product/1  "<AxlTrq>"
  scale factors with friction/1(lambdas) -> Combined Slip Wheel 2DOF/9
  Veh2Tire/5(psidot) -> Combined Slip Wheel 2DOF/5
  Combined Slip Wheel 2DOF/3 -> Tire2Veh/1(Fx)
  Combined Slip Wheel 2DOF/4 -> Tire2Veh/2(Fy)
  Combined Slip Wheel 2DOF/5 -> Tire2Veh/3(Fz)
  WhlAng/1 -> [WhlAng], Wheel Angles/1(steer)  "WhlAng"
  Gamma/1 -> [Gamma], Wheel Angles/2(camber)  "WhlCmb"
  Tire2Veh/1(FxyF) -> FrontF/1
  Tire2Veh/2(FxyR) -> RearF/1
  Veh2Tire/2(T) -> Combined Slip Wheel 2DOF/1
  BrkPrs/1 -> Veh2Tire/2(BrkPrs)
  AxlTrq/1 -> Veh2Tire/1(AxlTrq)
  Wheel Angles/1(WhlAngB) -> Veh2Tire/5(WhlAng)
  VehVel/1 -> Veh2Tire/4(VehVel)
  Veh2Tire/6(zdotAxle) -> Terminator2/1
  Veh2Tire/4(ydotAxle) -> Combined Slip Wheel 2DOF/3
  YawRate/1 -> Veh2Tire/3(r)
  [WhlAng] -> Tire2Veh/4(WhlAng)
  [Gamma] -> Combined Slip Wheel 2DOF/4
  [Gamma] -> Tire2Veh/5(WhlCmb)
  Veh2Tire/1(P) -> Terminator/1

== system Current_Macchina3DOF/Powertrain & Driveline/Driveline ==
  Gear : Inport
  TPowertrain : Inport  Port=2  PortDimensions=1
  AWD : Subsystem  VariantControl=2
  FWD : Subsystem  VariantControl=1
  RWD : Subsystem  VariantControl=0
  TAxles : Outport  PortDimensions=4  VectorParamsAs1DForOutWhenUnconnected=off

== system Current_Macchina3DOF/Powertrain & Driveline/Dual ==
  VehFdbk : Inport
  Dual Fz : Subsystem
  Dual V : Subsystem
  VehVel : Outport  VectorParamsAs1DForOutWhenUnconnected=off
  Fz : Outport  Port=2  VectorParamsAs1DForOutWhenUnconnected=off
  wires:
  Dual V/1(Out1) -> VehVel/1
  VehFdbk/1 -> Dual Fz/1(In1), Dual V/1(In1)
  Dual Fz/1(Out1) -> Fz/1

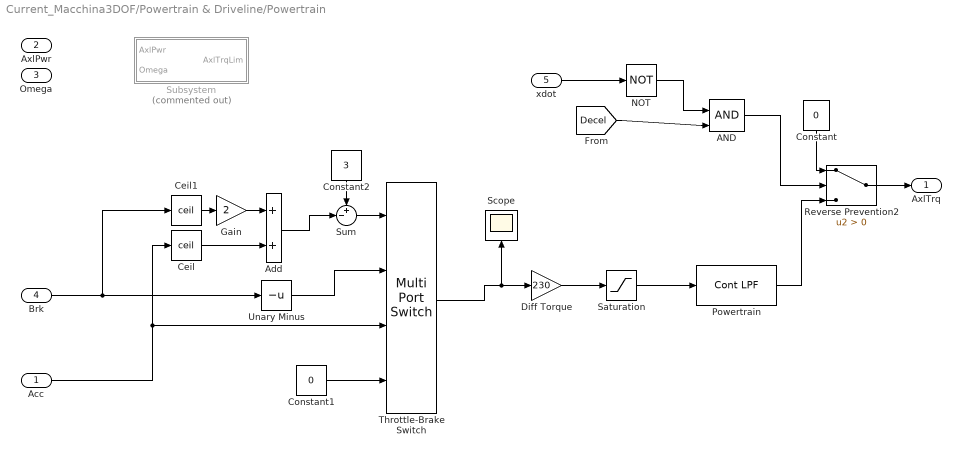
== system Current_Macchina3DOF/Powertrain & Driveline/Powertrain ==
  Acc : Inport
  AxlPwr : Inport  Port=2  PortDimensions=4
  Omega : Inport  Port=3  PortDimensions=4
  Brk : Inport  Port=4
  xdot : Inport  Port=5
  AND : Logic  IconShape=distinctive  AllPortsSameDT=off  OutDataTypeStr=boolean
  Add : Sum
  Ceil : Rounding  Operator=ceil
  Ceil1 : Rounding  Operator=ceil
  Constant : Constant  Value=0
  Constant1 : Constant  Value=0
  Constant2 : Constant  Value=3
  Diff Torque : Gain  Gain=230
  Gain : Gain  Gain=2
  NOT : Logic  Operator=NOT  IconShape=distinctive  AllPortsSameDT=off  OutDataTypeStr=boolean
  Powertrain : autolibutils/Cont LPF  wc=EngWc*2  AbsoluteTolerance=auto  aMode=2
  Reverse Prevention2 : Switch  Criteria=u2 > Threshold  SaturateOnIntegerOverflow=off  InputSameDT=off
  Saturation : Saturate  UpperLimit=230  LowerLimit=-230
  Scope : Scope
  Subsystem : Subsystem  Commented=on
  Sum : Sum  Inputs=+-|
  Throttle-Brake Switch : MultiPortSwitch  DiagnosticForDefault=None  SaturateOnIntegerOverflow=off  InputSameDT=off
  Unary Minus : UnaryMinus
  AxlTrq : Outport  VectorParamsAs1DForOutWhenUnconnected=off
  wires:
  Saturation/1 -> Powertrain/1
  Acc/1 -> Ceil/1, Throttle-Brake Switch/3
  Throttle-Brake Switch/1 -> Scope/1, Diff Torque/1
  Constant1/1 -> Throttle-Brake Switch/4
  Unary Minus/1 -> Throttle-Brake Switch/2
  Add/1 -> Sum/2
  Brk/1 -> Ceil1/1, Unary Minus/1
  Ceil/1 -> Add/2
  Ceil1/1 -> Gain/1
  Gain/1 -> Add/1
  Sum/1 -> Throttle-Brake Switch/1
  Constant2/1 -> Sum/1
  Diff Torque/1 -> Saturation/1
  Powertrain/1 -> Reverse Prevention2/3
  xdot/1 -> NOT/1
  NOT/1 -> AND/1
  AND/1 -> Reverse Prevention2/2
  Reverse Prevention2/1 -> AxlTrq/1
  Constant/1 -> Reverse Prevention2/1
  [Decel] -> AND/2

== system Current_Macchina3DOF/Powertrain & Driveline/Subsystem ==
  Mux : Mux  Inputs=3
  DriverCmd : Outport  VectorParamsAs1DForOutWhenUnconnected=off
  wires:
  [Decel] -> Mux/2
  Mux/1 -> DriverCmd/1
  [Acc] -> Mux/1
  [Gear] -> Mux/3

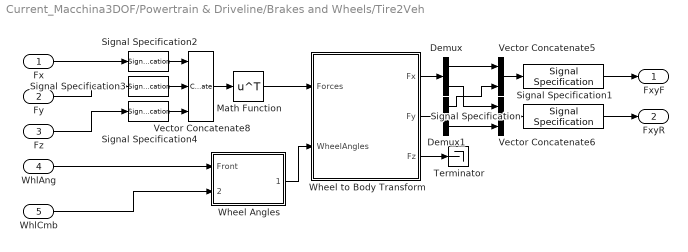
== system Current_Macchina3DOF/Powertrain & Driveline/Brakes and Wheels/Tire2Veh ==
  Fx : Inport
  Fy : Inport  Port=2
  Fz : Inport  Port=3
  WhlAng : Inport  Port=4
  WhlCmb : Inport  Port=5
  Demux : Demux  Outputs=[2,2]
  Demux1 : Demux  Outputs=[2,2]
  Math Function : Math  Operator=transpose  SignedPower=on
  Signal Specification : SignalSpecification  Unit=N
  Signal Specification1 : SignalSpecification  Unit=N
  Signal Specification2 : SignalSpecification  Dimensions=4
  Signal Specification3 : SignalSpecification  Dimensions=4
  Signal Specification4 : SignalSpecification  Dimensions=4
  Terminator : Terminator
  Vector Concatenate5 : Concatenate  Mode=Multidimensional array  ConcatenateDimension=2
  Vector Concatenate6 : Concatenate  Mode=Multidimensional array  ConcatenateDimension=2
  Vector Concatenate8 : Concatenate  NumInputs=3  Mode=Multidimensional array  ConcatenateDimension=2
  Wheel Angles : Subsystem
  Wheel to Body Transform : Subsystem
  FxyF : Outport
  FxyR : Outport  Port=2
  wires:
  Wheel Angles/1(Vehicle) -> Wheel to Body Transform/2(WheelAngles)
  Vector Concatenate5/1 -> Signal Specification1/1
  Demux/1 -> Vector Concatenate5/1
  Vector Concatenate8/1 -> Math Function/1
  Signal Specification1/1 -> FxyF/1
  Wheel to Body Transform/1(Fx) -> Demux/1
  Vector Concatenate6/1 -> Signal Specification/1
  Signal Specification4/1 -> Vector Concatenate8/3
  Demux1/2 -> Vector Concatenate6/2
  Wheel to Body Transform/2(Fy) -> Demux1/1
  Fy/1 -> Signal Specification3/1
  Math Function/1 -> Wheel to Body Transform/1(Forces)
  Wheel to Body Transform/3(Fz) -> Terminator/1
  Demux/2 -> Vector Concatenate6/1
  Signal Specification3/1 -> Vector Concatenate8/2
  Signal Specification2/1 -> Vector Concatenate8/1
  Demux1/1 -> Vector Concatenate5/2
  WhlAng/1 -> Wheel Angles/1(Front)
  Fx/1 -> Signal Specification2/1
  Fz/1 -> Signal Specification4/1
  Signal Specification/1 -> FxyR/1
  WhlCmb/1 -> Wheel Angles/2(Camber)

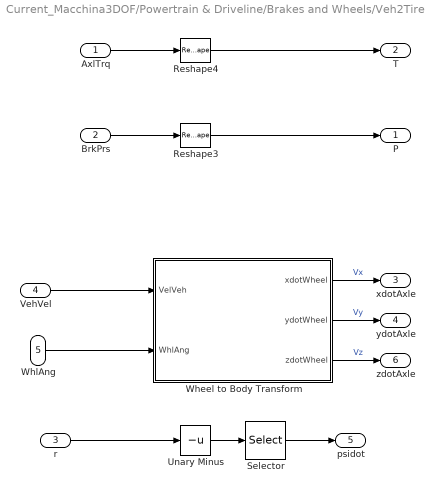
== system Current_Macchina3DOF/Powertrain & Driveline/Brakes and Wheels/Veh2Tire ==
  AxlTrq : Inport
  BrkPrs : Inport  Port=2
  r : Inport  Port=3
  VehVel : Inport  Port=4
  WhlAng : Inport  Port=5
  Reshape3 : Reshape
  Reshape4 : Reshape
  Selector : Selector  InputPortWidth=1  IndexOptions=Index vector (dialog)  Indices=[1 1 1 1]  OutputSizes=1
  Unary Minus : UnaryMinus
  Wheel to Body Transform : Subsystem
  P : Outport  VectorParamsAs1DForOutWhenUnconnected=off
  T : Outport  Port=2  VectorParamsAs1DForOutWhenUnconnected=off
  xdotAxle : Outport  Port=3  VectorParamsAs1DForOutWhenUnconnected=off
  ydotAxle : Outport  Port=4  VectorParamsAs1DForOutWhenUnconnected=off
  psidot : Outport  Port=5  VectorParamsAs1DForOutWhenUnconnected=off
  zdotAxle : Outport  Port=6  VectorParamsAs1DForOutWhenUnconnected=off
  wires:
  BrkPrs/1 -> Reshape3/1
  AxlTrq/1 -> Reshape4/1
  Wheel to Body Transform/1(xdotWheel) -> xdotAxle/1  "Vx"
  Wheel to Body Transform/2(ydotWheel) -> ydotAxle/1  "Vy"
  r/1 -> Unary Minus/1
  Reshape4/1 -> T/1
  VehVel/1 -> Wheel to Body Transform/1(VelVeh)
  Wheel to Body Transform/3(zdotWheel) -> zdotAxle/1  "Vz"
  Unary Minus/1 -> Selector/1
  Reshape3/1 -> P/1
  WhlAng/1 -> Wheel to Body Transform/2(WhlAng)
  Selector/1 -> psidot/1

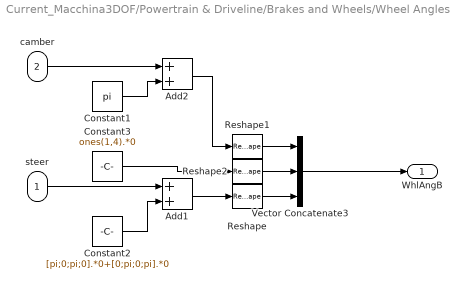
== system Current_Macchina3DOF/Powertrain & Driveline/Brakes and Wheels/Wheel Angles ==
  steer : Inport
  camber : Inport  Port=2
  Add1 : Sum
  Add2 : Sum
  Constant1 : Constant  Value=pi
  Constant2 : Constant  Value=[pi;0;pi;0].*0+[0;pi;0;pi].*0
  Constant3 : Constant  Value=ones(1,4).*0
  Reshape : Reshape  OutputDimensionality=Row vector (2-D)
  Reshape1 : Reshape  OutputDimensionality=Row vector (2-D)
  Reshape2 : Reshape  OutputDimensionality=Row vector (2-D)
  Vector Concatenate3 : Concatenate  NumInputs=3  Mode=Multidimensional array
  WhlAngB : Outport  VectorParamsAs1DForOutWhenUnconnected=off
  wires:
  Constant1/1 -> Add2/2
  Add2/1 -> Reshape1/1
  Add1/1 -> Reshape/1
  Reshape2/1 -> Vector Concatenate3/2
  Reshape1/1 -> Vector Concatenate3/1
  Constant3/1 -> Reshape2/1
  camber/1 -> Add2/1
  steer/1 -> Add1/1
  Reshape/1 -> Vector Concatenate3/3
  Vector Concatenate3/1 -> WhlAngB/1
  Constant2/1 -> Add1/2

== system Current_Macchina3DOF/Powertrain & Driveline/Brakes and Wheels/scale factors with friction ==
  lamda_mu_x : Inport
  lamda_mu_y : Inport  Port=2
  0 : Constant  Value=[zeros(1,numWheels)]  VectorParams1D=off
  Reshape : Reshape  OutputDimensionality=Row vector (2-D)  OutputDimensions=[1,numWheels]
  Reshape1 : Reshape  OutputDimensionality=Row vector (2-D)  OutputDimensions=[1,numWheels]
  Signal Specification3 : SignalSpecification  Unit=1
  Vector Concatenate : Concatenate  NumInputs=5  Mode=Multidimensional array
  ones : Constant  Value=[ones(23,numWheels)]  VectorParams1D=off
  ones2 : Constant  Value=ones(1,numWheels)  VectorParams1D=off
  lambdas : Outport  Unit=1  VectorParamsAs1DForOutWhenUnconnected=off
  wires:
  lamda_mu_y/1 -> Reshape1/1
  lamda_mu_x/1 -> Reshape/1
  ones2/1 -> Vector Concatenate/1  "lambda_Fz0"
  Vector Concatenate/1 -> Signal Specification3/1
  ones/1 -> Vector Concatenate/5
  0/1 -> Vector Concatenate/4  "lamda_mu_V"
  Reshape1/1 -> Vector Concatenate/3
  Reshape/1 -> Vector Concatenate/2
  Signal Specification3/1 -> lambdas/1

== system Current_Macchina3DOF/Powertrain & Driveline/Driveline/AWD ==
  TPowertrain : Inport
  Gear : Inport  Port=2
  AWD : Gain  Gain=[1;1;1;1]./2
  Add : Sum
  Constant : Constant
  Constant1 : Constant  Value=zeros(4,1)
  Multiport Switch : MultiPortSwitch  DataPortOrder=Zero-based contiguous  zeroidx=on  SaturateOnIntegerOverflow=off  InputSameDT=off
  Unary Minus : UnaryMinus
  TAxles : Outport  VectorParamsAs1DForOutWhenUnconnected=off
  wires:
  TPowertrain/1 -> AWD/1
  Multiport Switch/1 -> TAxles/1
  Add/1 -> Multiport Switch/1
  Constant1/1 -> Multiport Switch/3
  AWD/1 -> Unary Minus/1, Multiport Switch/4
  Constant/1 -> Add/2
  Gear/1 -> Add/1
  Unary Minus/1 -> Multiport Switch/2

== system Current_Macchina3DOF/Powertrain & Driveline/Driveline/FWD ==
  TPowertrain : Inport
  Gear : Inport  Port=2
  Add : Sum
  Constant : Constant
  Constant1 : Constant  Value=zeros(4,1)
  FWD : Gain  Gain=[1;1;0;0]
  Multiport Switch : MultiPortSwitch  DataPortOrder=Zero-based contiguous  zeroidx=on  SaturateOnIntegerOverflow=off  InputSameDT=off
  Unary Minus : UnaryMinus
  TAxles : Outport  VectorParamsAs1DForOutWhenUnconnected=off
  wires:
  TPowertrain/1 -> FWD/1
  Multiport Switch/1 -> TAxles/1
  Add/1 -> Multiport Switch/1
  Constant1/1 -> Multiport Switch/3
  FWD/1 -> Unary Minus/1, Multiport Switch/4
  Constant/1 -> Add/2
  Gear/1 -> Add/1
  Unary Minus/1 -> Multiport Switch/2

== system Current_Macchina3DOF/Powertrain & Driveline/Driveline/RWD ==
  TPowertrain : Inport
  Gear : Inport  Port=2
  Add : Sum
  Constant : Constant
  Constant1 : Constant  Value=zeros(4,1)
  Multiport Switch : MultiPortSwitch  DataPortOrder=Zero-based contiguous  zeroidx=on  SaturateOnIntegerOverflow=off  InputSameDT=off
  RWD : Gain  Gain=[0;0;1.4;1.4]
  Unary Minus : UnaryMinus
  TAxles : Outport  VectorParamsAs1DForOutWhenUnconnected=off
  wires:
  RWD/1 -> Unary Minus/1, Multiport Switch/4
  TPowertrain/1 -> RWD/1
  Unary Minus/1 -> Multiport Switch/2
  Multiport Switch/1 -> TAxles/1
  Gear/1 -> Add/1
  Constant/1 -> Add/2
  Add/1 -> Multiport Switch/1
  Constant1/1 -> Multiport Switch/3

== system Current_Macchina3DOF/Powertrain & Driveline/Dual/Dual Fz ==
  In1 : Inport
  Add : Sum
  Bus Selector6 : BusSelector  OutputSignals=BdyFrm.Forces.Tires.FrntTires.Lft.Fz,BdyFrm.Forces.Tires.FrntTires.Rght.Fz,BdyFrm.Forces.Tires.RearTires.Lft.Fz,BdyFrm.Forces.Tires.RearTires.Rght.Fz
  Cont LPF : autolibutils/Cont LPF  wc=100*2*pi  AbsoluteTolerance=auto  aMode=2
  Saturation : Saturate  UpperLimit=10e3  LowerLimit=100  ZeroCross=off
  Unsprung Mass : Constant  Value=[0 0 80 80].*9.81
  Vector Concatenate : Concatenate  NumInputs=4
  Out1 : Outport  VectorParamsAs1DForOutWhenUnconnected=off
  wires:
  Saturation/1 -> Cont LPF/1
  Cont LPF/1 -> Add/1
  Vector Concatenate/1 -> Saturation/1
  Bus Selector6/2 -> Vector Concatenate/2  "<Fz>"
  Bus Selector6/1 -> Vector Concatenate/1  "<Fz>"
  Bus Selector6/3 -> Vector Concatenate/3  "<Fz>"
  Bus Selector6/4 -> Vector Concatenate/4  "<Fz>"
  Add/1 -> Out1/1
  Unsprung Mass/1 -> Add/2
  In1/1 -> Bus Selector6/1

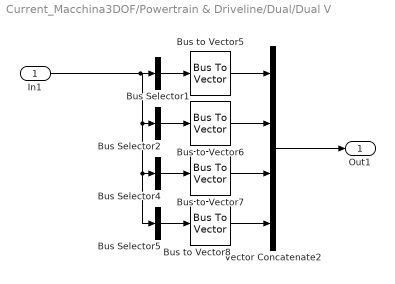
== system Current_Macchina3DOF/Powertrain & Driveline/Dual/Dual V ==
  In1 : Inport
  Bus Selector1 : BusSelector  OutputSignals=BdyFrm.FrntAxl.Lft.Vel.xdot,BdyFrm.FrntAxl.Lft.Vel.ydot,BdyFrm.FrntAxl.Lft.Vel.zdot  OutputAsBus=on
  Bus Selector2 : BusSelector  OutputSignals=BdyFrm.FrntAxl.Rght.Vel.xdot,BdyFrm.FrntAxl.Rght.Vel.ydot,BdyFrm.FrntAxl.Rght.Vel.zdot  OutputAsBus=on
  Bus Selector4 : BusSelector  OutputSignals=BdyFrm.RearAxl.Lft.Vel.xdot,BdyFrm.RearAxl.Lft.Vel.ydot,BdyFrm.RearAxl.Lft.Vel.zdot  OutputAsBus=on
  Bus Selector5 : BusSelector  OutputSignals=BdyFrm.RearAxl.Rght.Vel.xdot,BdyFrm.RearAxl.Rght.Vel.ydot,BdyFrm.RearAxl.Rght.Vel.zdot  OutputAsBus=on
  Bus to Vector{5..8} (4 alike) : BusToVector
  Vector Concatenate2 : Concatenate  NumInputs=4  Mode=Multidimensional array  ConcatenateDimension=2
  Out1 : Outport  VectorParamsAs1DForOutWhenUnconnected=off
  wires:
  Bus to Vector6/1 -> Vector Concatenate2/2
  Bus Selector2/1 -> Bus to Vector6/1
  Bus to Vector8/1 -> Vector Concatenate2/4
  Bus Selector4/1 -> Bus to Vector7/1
  Bus to Vector5/1 -> Vector Concatenate2/1
  Bus Selector1/1 -> Bus to Vector5/1
  In1/1 -> Bus Selector1/1, Bus Selector2/1, Bus Selector4/1, Bus Selector5/1
  Bus Selector5/1 -> Bus to Vector8/1
  Bus to Vector7/1 -> Vector Concatenate2/3
  Vector Concatenate2/1 -> Out1/1

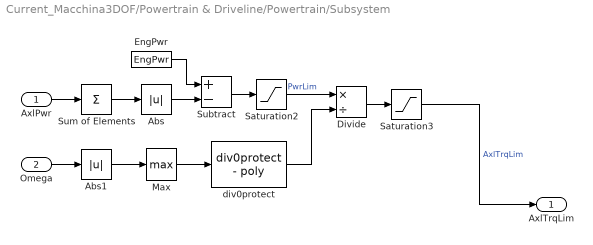
== system Current_Macchina3DOF/Powertrain & Driveline/Powertrain/Subsystem ==
  AxlPwr : Inport  PortDimensions=4
  Omega : Inport  Port=2  PortDimensions=4
  Abs : Abs  ZeroCross=off  SaturateOnIntegerOverflow=off
  Abs1 : Abs  ZeroCross=off  SaturateOnIntegerOverflow=off
  Divide : Product  Inputs=*/
  EngPwr : Constant  Value=EngPwr
  Max : MinMax  Function=max  ZeroCross=off
  Saturation2 : Saturate  UpperLimit=inf  LowerLimit=100  ZeroCross=off
  Saturation3 : Saturate  UpperLimit=Tlim  LowerLimit=0  ZeroCross=off
  Subtract : Sum  Inputs=+-
  Sum of Elements : Sum  Inputs=+
  div0protect : autolibutils/div0protect - poly  thresh=1  ZeroCross1=on  aMode=2
  AxlTrqLim : Outport
  wires:
  Sum of Elements/1 -> Abs/1
  div0protect/1 -> Divide/2
  Subtract/1 -> Saturation2/1
  Abs/1 -> Subtract/2
  Saturation2/1 -> Divide/1  "PwrLim"
  Divide/1 -> Saturation3/1
  Omega/1 -> Abs1/1
  Abs1/1 -> Max/1
  Max/1 -> div0protect/1
  AxlPwr/1 -> Sum of Elements/1
  EngPwr/1 -> Subtract/1
  Saturation3/1 -> AxlTrqLim/1  "AxlTrqLim"

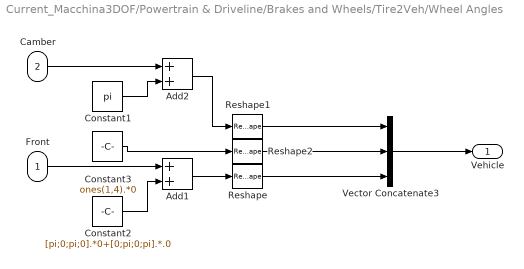
== system Current_Macchina3DOF/Powertrain & Driveline/Brakes and Wheels/Tire2Veh/Wheel Angles ==
  Front : Inport
  Camber : Inport  Port=2
  Add1 : Sum
  Add2 : Sum
  Constant1 : Constant  Value=pi
  Constant2 : Constant  Value=[pi;0;pi;0].*0+[0;pi;0;pi].*.0
  Constant3 : Constant  Value=ones(1,4).*0
  Reshape : Reshape  OutputDimensionality=Row vector (2-D)
  Reshape1 : Reshape  OutputDimensionality=Row vector (2-D)
  Reshape2 : Reshape  OutputDimensionality=Row vector (2-D)
  Vector Concatenate3 : Concatenate  NumInputs=3  Mode=Multidimensional array
  Vehicle : Outport  VectorParamsAs1DForOutWhenUnconnected=off
  wires:
  Constant1/1 -> Add2/2
  Reshape/1 -> Vector Concatenate3/3
  Reshape2/1 -> Vector Concatenate3/2
  Front/1 -> Add1/1
  Add2/1 -> Reshape1/1
  Add1/1 -> Reshape/1
  Constant3/1 -> Reshape2/1
  Reshape1/1 -> Vector Concatenate3/1
  Constant2/1 -> Add1/2
  Camber/1 -> Add2/1
  Vector Concatenate3/1 -> Vehicle/1

== system Current_Macchina3DOF/Powertrain & Driveline/Brakes and Wheels/Tire2Veh/Wheel to Body Transform ==
  Forces : Inport  PortDimensions=[3,1]  Partition=on  PartitionDimension=2  PartitionWidth=1  PartitionOffset=0
  WheelAngles : Inport  Port=2  Partition=on  PartitionDimension=2  PartitionWidth=1  PartitionOffset=0
  Demux1 : Demux  Outputs=3
  Divide1 : Product  Inputs=**  Multiplication=Matrix(*)
  For Each : ForEach  DisableCoverage=on
  Rotation Angles to Direction Cosine Matrix : sharedtransform/Rotation Angles to Direction Cosine Matrix  rotationOrder=ZYX  aMode=2
  Selector : Selector  InputPortWidth=3  IndexOptions=Index vector (dialog)  Indices=[3 2 1]  OutputSizes=1
  Fx : Outport  ConcatenationDimension=1  VectorParamsAs1DForOutWhenUnconnected=off
  Fy : Outport  Port=2  ConcatenationDimension=1  VectorParamsAs1DForOutWhenUnconnected=off
  Fz : Outport  Port=3  ConcatenationDimension=1  VectorParamsAs1DForOutWhenUnconnected=off
  wires:
  Divide1/1 -> Demux1/1
  Demux1/1 -> Fx/1
  Demux1/2 -> Fy/1
  Demux1/3 -> Fz/1
  Rotation Angles to Direction Cosine Matrix/1 -> Divide1/1
  Forces/1 -> Divide1/2
  WheelAngles/1 -> Selector/1
  Selector/1 -> Rotation Angles to Direction Cosine Matrix/1

== system Current_Macchina3DOF/Powertrain & Driveline/Brakes and Wheels/Veh2Tire/Wheel to Body Transform ==
  VelVeh : Inport  Partition=on  PartitionDimension=2  PartitionWidth=1  PartitionOffset=0
  WhlAng : Inport  Port=2  Partition=on  PartitionDimension=2  PartitionWidth=1  PartitionOffset=0
  Demux1 : Demux  Outputs=3
  Divide1 : Product  Inputs=**  Multiplication=Matrix(*)
  For Each : ForEach  DisableCoverage=on
  Rotation Angles to Direction Cosine Matrix : sharedtransform/Rotation Angles to Direction Cosine Matrix  rotationOrder=ZYX  aMode=2
  Selector : Selector  InputPortWidth=3  IndexOptions=Index vector (dialog)  Indices=[3 2 1]  OutputSizes=1
  xdotWheel : Outport  ConcatenationDimension=1  VectorParamsAs1DForOutWhenUnconnected=off
  ydotWheel : Outport  Port=2  ConcatenationDimension=1  VectorParamsAs1DForOutWhenUnconnected=off
  zdotWheel : Outport  Port=3  ConcatenationDimension=1  VectorParamsAs1DForOutWhenUnconnected=off
  wires:
  Divide1/1 -> Demux1/1
  Demux1/1 -> xdotWheel/1
  Demux1/2 -> ydotWheel/1
  Demux1/3 -> zdotWheel/1
  Rotation Angles to Direction Cosine Matrix/1 -> Divide1/1
  VelVeh/1 -> Divide1/2
  WhlAng/1 -> Selector/1
  Selector/1 -> Rotation Angles to Direction Cosine Matrix/1
